simulink model "gm_HA_sys8_vnl"  (R2018a)
settings: Solver=FixedStepDiscrete  StartTime=0.0  StopTime=stopTime  RelTol=1e-3
InitFcn:
  | HA_sys8_init
StopFcn:
  | HA_sys8_freq_response
undefined symbols (not defined in the file or in its folder): dspDeleteFVToolLinkFromMask, FIRBandPass1, FIRBandPass2, FIRBandPass3, FIRBandPass4, FIRDecimator1, FIRDecimator2, FIRDecimator3, FIRDecimator4, FIRInterpolator1, FIRInterpolator2, FIRInterpolator3, FIRInterpolator4, Fs, Gain_B1_left, Gain_B1_right, Gain_B2_left, Gain_B2_right, Gain_B3_left, Gain_B3_right, Gain_B4_left, Gain_B4_right, Gain_left_all, Gain_right_all, gcbh
libraries: hdlsllib x40, dspmlti4 x32, simulink x4, dspsrcs4 x1
(part 4 of 4)

== system gm_HA_sys8_vnl/HA_LR/HA_right/FIRInterpolator1 ==
  In1 : Inport
  FIRInterpolator1 : dspmlti4/FIR Interpolation  FilterSource=Dialog parameters  h=FIRInterpolator1.FIR_coefficients  L=FIRInterpolator1.interpolation_factor  FilterObject=FINTERP  framing=Allow multirate processing  outputBufInitCond=0  roundingMode=Floor  overflowMode=on  firstCoeffDataTypeStr=Inherit: Same word length as input  firstCoeffMin=[]  firstCoeffMax=[]  firstCoeffLastDataTypeStr=Inherit: Same word length as input  outputMode=Binary point scaling  outputWordLength=32  outputFracLength=28  outputDataTypeStr=fixdt(1,32,28)  outputMin=[]  outputMax=[]  outputLastDataTypeStr=fixdt(1,32,28)
      settings: SourceProductName=DSP System Toolbox
  FIRInterpolator1_GenDelay1 : Delay  DelayLength=1  InputProcessing=Inherited
  Out1 : Outport
  wires:
  FIRInterpolator1_GenDelay1/1 -> Out1/1
  FIRInterpolator1/1 -> FIRInterpolator1_GenDelay1/1
  In1/1 -> FIRInterpolator1/1

== system gm_HA_sys8_vnl/HA_LR/HA_right/FIRInterpolator2 ==
  In1 : Inport
  FIRInterpolator2 : dspmlti4/FIR Interpolation  FilterSource=Dialog parameters  h=FIRInterpolator2.FIR_coefficients  L=FIRInterpolator2.interpolation_factor  FilterObject=FINTERP  framing=Allow multirate processing  outputBufInitCond=0  roundingMode=Floor  overflowMode=on  firstCoeffDataTypeStr=Inherit: Same word length as input  firstCoeffMin=[]  firstCoeffMax=[]  firstCoeffLastDataTypeStr=Inherit: Same word length as input  outputMode=Binary point scaling  outputWordLength=32  outputFracLength=28  outputDataTypeStr=fixdt(1,32,28)  outputMin=[]  outputMax=[]  outputLastDataTypeStr=fixdt(1,32,28)
      settings: SourceProductName=DSP System Toolbox
  FIRInterpolator2_GenDelay1 : Delay  DelayLength=1  InputProcessing=Inherited
  Out1 : Outport
  wires:
  FIRInterpolator2_GenDelay1/1 -> Out1/1
  FIRInterpolator2/1 -> FIRInterpolator2_GenDelay1/1
  In1/1 -> FIRInterpolator2/1

== system gm_HA_sys8_vnl/HA_LR/HA_right/FIRInterpolator3 ==
  In1 : Inport
  FIRInterpolator3 : dspmlti4/FIR Interpolation  FilterSource=Dialog parameters  h=FIRInterpolator3.FIR_coefficients  L=FIRInterpolator3.interpolation_factor  FilterObject=FINTERP  framing=Allow multirate processing  outputBufInitCond=0  roundingMode=Floor  overflowMode=on  firstCoeffDataTypeStr=Inherit: Same word length as input  firstCoeffMin=[]  firstCoeffMax=[]  firstCoeffLastDataTypeStr=Inherit: Same word length as input  outputMode=Binary point scaling  outputWordLength=32  outputFracLength=28  outputDataTypeStr=fixdt(1,32,28)  outputMin=[]  outputMax=[]  outputLastDataTypeStr=fixdt(1,32,28)
      settings: SourceProductName=DSP System Toolbox
  FIRInterpolator3_GenDelay1 : Delay  DelayLength=1  InputProcessing=Inherited
  Out1 : Outport
  wires:
  FIRInterpolator3_GenDelay1/1 -> Out1/1
  FIRInterpolator3/1 -> FIRInterpolator3_GenDelay1/1
  In1/1 -> FIRInterpolator3/1

== system gm_HA_sys8_vnl/HA_LR/HA_right/FIRInterpolator4 ==
  In1 : Inport
  FIRInterpolator4 : dspmlti4/FIR Interpolation  FilterSource=Dialog parameters  h=FIRInterpolator4.FIR_coefficients  L=FIRInterpolator4.interpolation_factor  FilterObject=FINTERP  framing=Allow multirate processing  outputBufInitCond=0  roundingMode=Floor  overflowMode=on  firstCoeffDataTypeStr=Inherit: Same word length as input  firstCoeffMin=[]  firstCoeffMax=[]  firstCoeffLastDataTypeStr=Inherit: Same word length as input  outputMode=Binary point scaling  outputWordLength=32  outputFracLength=28  outputDataTypeStr=fixdt(1,32,28)  outputMin=[]  outputMax=[]  outputLastDataTypeStr=fixdt(1,32,28)
      settings: SourceProductName=DSP System Toolbox
  FIRInterpolator4_GenDelay1 : Delay  DelayLength=1  InputProcessing=Inherited
  Out1 : Outport
  wires:
  FIRInterpolator4_GenDelay1/1 -> Out1/1
  FIRInterpolator4/1 -> FIRInterpolator4_GenDelay1/1
  In1/1 -> FIRInterpolator4/1
